simulink model "controlSistem"  (R2016b)
settings: Solver=VariableStepAuto  StartTime=0.0  StopTime=200.0  RelTol=1e-3
libraries: fuzblock x1
settings Model: Creator=novo  LastModifiedBy=novo
settings SolverCC: ZeroCrossAlgorithm=Adaptive

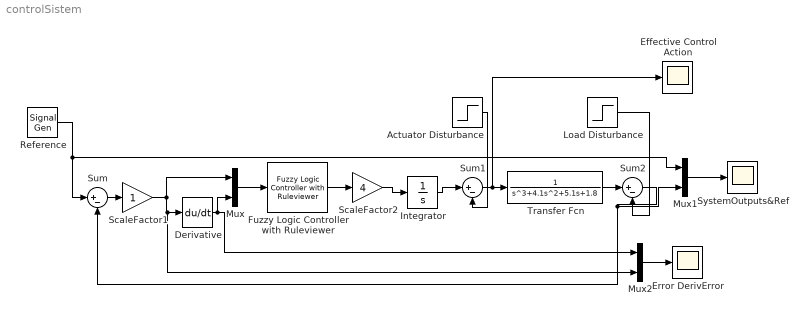
== system controlSistem ==
  Actuator Disturbance : Step  Time=100  SampleTime=0
  Derivative : Derivative
  Effective Control Action : Scope
  Error DerivError : Scope
  Fuzzy Logic Controller with Ruleviewer : fuzblock/Fuzzy Logic  Controller  with Ruleviewer  fismatrix=sugeno25rules  Ts=2
  Integrator : Integrator
  Load Disturbance : Step  Time=190  SampleTime=0
  Mux : Mux  Inputs=2
  Mux1 : Mux  Inputs=2
  Mux2 : Mux  Inputs=2
  Reference : SignalGenerator  WaveForm=square  Amplitude=0.5  Frequency=0.1  Units=rad/sec
  ScaleFactor1 : Gain
  ScaleFactor2 : Gain  Gain=4
  Sum : Sum  Inputs=|+-
  Sum1 : Sum  Inputs=|+-
  Sum2 : Sum  Inputs=|+-
  SystemOutputs&Ref : Scope
  Transfer Fcn : TransferFcn  Denominator=[1 4.1 5.1 1.8]
  wires:
  Reference/1 -> Mux1/1, Sum/1
  ScaleFactor1/1 -> Mux/1, Mux2/2, Derivative/1
  Sum/1 -> ScaleFactor1/1
  Derivative/1 -> Mux2/1, Mux/2
  Mux/1 -> Fuzzy Logic Controller with Ruleviewer/1
  ScaleFactor2/1 -> Integrator/1
  Fuzzy Logic Controller with Ruleviewer/1 -> ScaleFactor2/1
  Integrator/1 -> Sum1/1
  Sum1/1 -> Effective Control Action/1, Transfer Fcn/1
  Transfer Fcn/1 -> Sum2/1
  Sum2/1 -> Mux1/2, Sum/2
  Actuator Disturbance/1 -> Sum1/2
  Load Disturbance/1 -> Sum2/2
  Mux1/1 -> SystemOutputs&Ref/1
  Mux2/1 -> Error DerivError/1
